simulink model "SecRwRtStLgrstUpwdDnwdCtrl"  (R2018b)
settings: Solver=FixedStepDiscrete  StartTime=0.0  StopTime=10.0  FixedStep=0.01  RelTol=1e-3
undefined symbols (not defined in the file or in its folder): KeSMSuMdMotFinshdTm_Val, KeSMSuMdRetryTm1_Val, KeSMSuModeReqDurgTm_Val, KeSMSwSecRwRtStLgrstUpwdDnwdEnTrigBitMask_Val
libraries: StCtrlLibBkRecln x1
settings Model: Creator=sn2xws  LastModifiedBy=sn55gm
settings Model: ModifiedHistory=|
  | 2024.10.14 V3.0.0 bitmask 更换变量接口
  | 25.7.7 V3.13.0 Md61 Md62新增Retry口
settings DataIOCC: SaveFormat=StructureWithTime
settings OptimizationCC: DefaultParameterBehavior=Inlined  EnhancedBackFolding=on  PassReuseOutputArgsAs=Individual arguments  ZeroExternalMemoryAtStartup=off  ZeroInternalMemoryAtStartup=off  OptimizeBlockOrder=speed  DifferentSizesBufferReuse=on  OptimizationCustomize=off
settings DebuggingCC: ParameterTunabilityLossMsg=error
settings ModelReferenceCC: ModelReferenceNumInstancesAllowed=Single
settings SFSimCC: MATLABDynamicMemAlloc=off
settings RTWCC: SystemTargetFile=autosar.tlc  GenCodeOnly=on  TemplateMakefile=ert_default_tmf  Description=AUTOSAR  GenerateReport=on  IncludeHyperlinkInReport=on  LaunchReport=on  GenerateTraceInfo=on  GenerateTraceReport=on  GenerateTraceReportSl=on  GenerateTraceReportSf=on  GenerateTraceReportEml=on
settings CodeAppCC: ForceParamTrailComments=on  IgnoreCustomStorageClasses=off  OperatorAnnotations=on  SimulinkDataObjDesc=on  SFDataObjDesc=on  InsertBlockDesc=on
settings STFCustomTargetCC: TargetLangStandard=C99 (ISO)  MultiwordLength=256  ParMdlRefBuildCompliant=on  CompOptLevelCompliant=on  IncludeMdlTerminateFcn=off  CombineOutputUpdateFcns=on  SuppressErrorStatus=on  ERTCustomFileBanners=on  SupportNonFinite=off  SupportComplex=off  SupportContinuousTime=off  SupportNonInlinedSFcns=off  RemoveResetFunc=on  MATLABClassNameForMDSCustomization=Simulink.SoftwareTarget.ERTCustomization  AutosarCompliant=on  UseToolchainInfoCompliant=on  LookupTableObjectStructAxisOrder=2,1,3,4,...  LUTObjectStructOrderEvenSpacing=Size,Table,Breakpoints  SystemTargetFile=autosar.tlc
settings ERTTargetCC: TargetLangStandard=C99 (ISO)  ConcurrentExecutionCompliant=off  IncludeMdlTerminateFcn=off  SuppressErrorStatus=on  SupportNonFinite=off  SupportComplex=off  ModelStepFunctionPrototypeControlCompliant=off  CPPClassGenCompliant=off  AutosarCompliant=on  LookupTableObjectStructAxisOrder=2,1,3,4,...  LUTObjectStructOrderEvenSpacing=Size,Table,Breakpoints  InlinedParameterPlacement=NonHierarchical  ERTCustomFileTemplate=example_file_process.tlc  ERTFilePackagingFormat=Compact

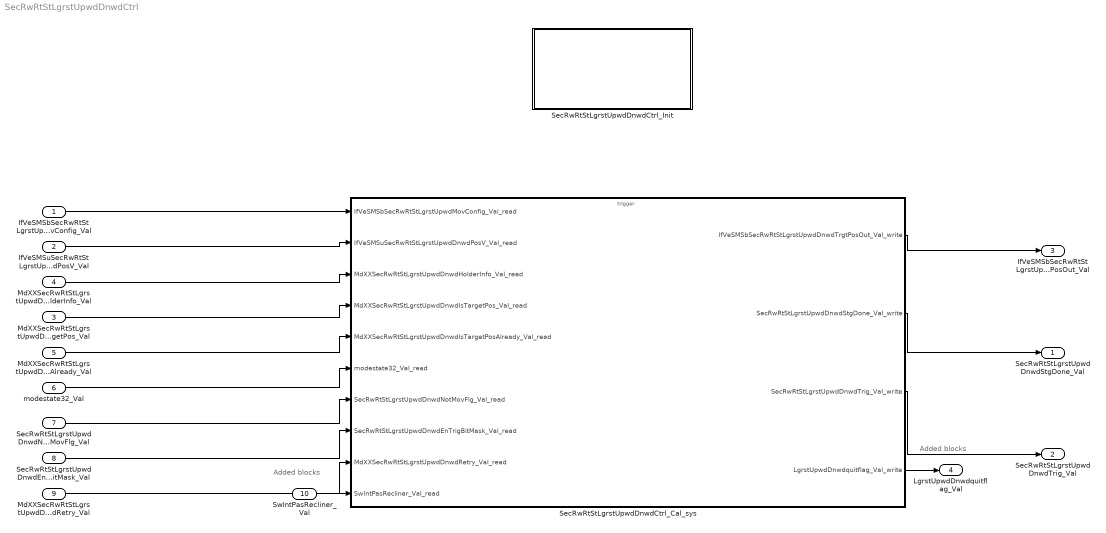
== system SecRwRtStLgrstUpwdDnwdCtrl ==
  note: Added blocks
  note: Added blocks
  IfVeSMSbSecRwRtStLgrstUpwdMovConfig_Val : Inport  OutDataTypeStr=boolean  PortDimensions=1
  IfVeSMSuSecRwRtStLgrstUpwdDnwdPosV_Val : Inport  Port=2  OutDataTypeStr=boolean  PortDimensions=1
  MdXXSecRwRtStLgrstUpwdDnwdIsTargetPos_Val : Inport  Port=3  OutDataTypeStr=uint32  PortDimensions=1
  MdXXSecRwRtStLgrstUpwdDnwdHolderInfo_Val : Inport  Port=4  OutDataTypeStr=uint32  PortDimensions=1
  MdXXSecRwRtStLgrstUpwdDnwdIsTargetPosAlready_Val : Inport  Port=5  OutDataTypeStr=uint32  PortDimensions=1
  modestate32_Val : Inport  Port=6  OutDataTypeStr=uint32  PortDimensions=1
  SecRwRtStLgrstUpwdDnwdNotMovFlg_Val : Inport  Port=7  OutDataTypeStr=boolean  PortDimensions=1
  SecRwRtStLgrstUpwdDnwdEnTrigBitMask_Val : Inport  Port=8  OutDataTypeStr=uint32  PortDimensions=1
  MdXXSecRwRtStLgrstUpwdDnwdRetry_Val : Inport  Port=9  OutDataTypeStr=uint32  PortDimensions=1
  SwIntPasRecliner_Val : Inport  Port=10  OutDataTypeStr=boolean  PortDimensions=1
  SecRwRtStLgrstUpwdDnwdCtrl_Cal_sys : Subsystem
  SecRwRtStLgrstUpwdDnwdCtrl_Init : Subsystem
  SecRwRtStLgrstUpwdDnwdStgDone_Val : Outport  OutDataTypeStr=boolean  PortDimensions=1
  SecRwRtStLgrstUpwdDnwdTrig_Val : Outport  Port=2  OutDataTypeStr=boolean  PortDimensions=1
  IfVeSMSbSecRwRtStLgrstUpwdDnwdTrgtPosOut_Val : Outport  Port=3  OutDataTypeStr=boolean  PortDimensions=1
  LgrstUpwdDnwdquitflag_Val : Outport  Port=4  OutDataTypeStr=boolean  PortDimensions=1
  wires:
  IfVeSMSbSecRwRtStLgrstUpwdMovConfig_Val/1 -> SecRwRtStLgrstUpwdDnwdCtrl_Cal_sys/1(IfVeSMSbSecRwRtStLgrstUpwdMovConfig_Val_read)
  IfVeSMSuSecRwRtStLgrstUpwdDnwdPosV_Val/1 -> SecRwRtStLgrstUpwdDnwdCtrl_Cal_sys/2(IfVeSMSuSecRwRtStLgrstUpwdDnwdPosV_Val_read)
  MdXXSecRwRtStLgrstUpwdDnwdIsTargetPos_Val/1 -> SecRwRtStLgrstUpwdDnwdCtrl_Cal_sys/4(MdXXSecRwRtStLgrstUpwdDnwdIsTargetPos_Val_read)
  MdXXSecRwRtStLgrstUpwdDnwdHolderInfo_Val/1 -> SecRwRtStLgrstUpwdDnwdCtrl_Cal_sys/3(MdXXSecRwRtStLgrstUpwdDnwdHolderInfo_Val_read)
  MdXXSecRwRtStLgrstUpwdDnwdIsTargetPosAlready_Val/1 -> SecRwRtStLgrstUpwdDnwdCtrl_Cal_sys/5(MdXXSecRwRtStLgrstUpwdDnwdIsTargetPosAlready_Val_read)
  modestate32_Val/1 -> SecRwRtStLgrstUpwdDnwdCtrl_Cal_sys/6(modestate32_Val_read)
  SecRwRtStLgrstUpwdDnwdNotMovFlg_Val/1 -> SecRwRtStLgrstUpwdDnwdCtrl_Cal_sys/7(SecRwRtStLgrstUpwdDnwdNotMovFlg_Val_read)
  SecRwRtStLgrstUpwdDnwdCtrl_Cal_sys/1(IfVeSMSbSecRwRtStLgrstUpwdDnwdTrgtPosOut_Val_write) -> IfVeSMSbSecRwRtStLgrstUpwdDnwdTrgtPosOut_Val/1
  SecRwRtStLgrstUpwdDnwdCtrl_Cal_sys/2(SecRwRtStLgrstUpwdDnwdStgDone_Val_write) -> SecRwRtStLgrstUpwdDnwdStgDone_Val/1
  SecRwRtStLgrstUpwdDnwdCtrl_Cal_sys/3(SecRwRtStLgrstUpwdDnwdTrig_Val_write) -> SecRwRtStLgrstUpwdDnwdTrig_Val/1
  SecRwRtStLgrstUpwdDnwdEnTrigBitMask_Val/1 -> SecRwRtStLgrstUpwdDnwdCtrl_Cal_sys/8(SecRwRtStLgrstUpwdDnwdEnTrigBitMask_Val_read)
  MdXXSecRwRtStLgrstUpwdDnwdRetry_Val/1 -> SecRwRtStLgrstUpwdDnwdCtrl_Cal_sys/9(MdXXSecRwRtStLgrstUpwdDnwdRetry_Val_read)
  SecRwRtStLgrstUpwdDnwdCtrl_Cal_sys/4(LgrstUpwdDnwdquitflag_Val_write) -> LgrstUpwdDnwdquitflag_Val/1
  SwIntPasRecliner_Val/1 -> SecRwRtStLgrstUpwdDnwdCtrl_Cal_sys/10(SwIntPasRecliner_Val_read)

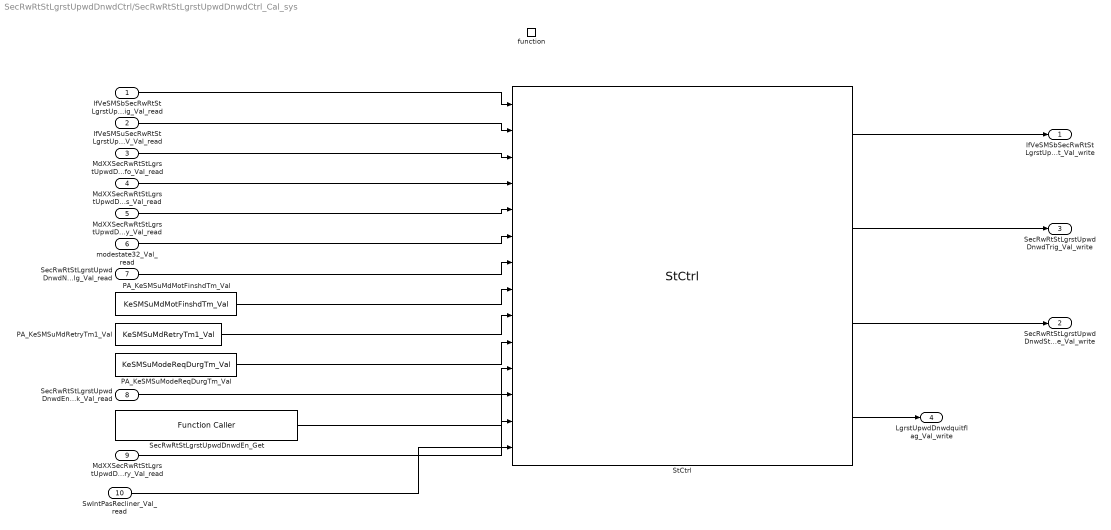
== system SecRwRtStLgrstUpwdDnwdCtrl/SecRwRtStLgrstUpwdDnwdCtrl_Cal_sys ==
  IfVeSMSbSecRwRtStLgrstUpwdMovConfig_Val_read : Inport
  IfVeSMSuSecRwRtStLgrstUpwdDnwdPosV_Val_read : Inport  Port=2
  MdXXSecRwRtStLgrstUpwdDnwdHolderInfo_Val_read : Inport  Port=3
  MdXXSecRwRtStLgrstUpwdDnwdIsTargetPos_Val_read : Inport  Port=4
  MdXXSecRwRtStLgrstUpwdDnwdIsTargetPosAlready_Val_read : Inport  Port=5
  modestate32_Val_read : Inport  Port=6
  SecRwRtStLgrstUpwdDnwdNotMovFlg_Val_read : Inport  Port=7
  SecRwRtStLgrstUpwdDnwdEnTrigBitMask_Val_read : Inport  Port=8
  MdXXSecRwRtStLgrstUpwdDnwdRetry_Val_read : Inport  Port=9
  SwIntPasRecliner_Val_read : Inport  Port=10
  function : TriggerPort  TriggerType=function-call  IsSimulinkFunction=on  FunctionName=SecRwRtStLgrstUpwdDnwdCtrl_Cal  VariantControl=(inherit)
  PA_KeSMSuMdMotFinshdTm_Val : Constant  Value=KeSMSuMdMotFinshdTm_Val
  PA_KeSMSuMdRetryTm1_Val : Constant  Value=KeSMSuMdRetryTm1_Val
  PA_KeSMSuModeReqDurgTm_Val : Constant  Value=KeSMSuModeReqDurgTm_Val
  SecRwRtStLgrstUpwdDnwdEn_Get : FunctionCaller  FunctionPrototype=data = SecRwRtStLgrstUpwdDnwdEn_Get()  OutputArgumentSpecifications=uint32(1)
  StCtrl : StCtrlLibBkRecln/StCtrl  SystemSampleTime=-1
  IfVeSMSbSecRwRtStLgrstUpwdDnwdTrgtPosOut_Val_write : Outport
      settings: EnsureOutportIsVirtual=on
  SecRwRtStLgrstUpwdDnwdStgDone_Val_write : Outport  Port=2
      settings: EnsureOutportIsVirtual=on
  SecRwRtStLgrstUpwdDnwdTrig_Val_write : Outport  Port=3
      settings: EnsureOutportIsVirtual=on
  LgrstUpwdDnwdquitflag_Val_write : Outport  Port=4
      settings: EnsureOutportIsVirtual=on
  wires:
  StCtrl/3 -> SecRwRtStLgrstUpwdDnwdStgDone_Val_write/1
  StCtrl/2 -> SecRwRtStLgrstUpwdDnwdTrig_Val_write/1
  StCtrl/1 -> IfVeSMSbSecRwRtStLgrstUpwdDnwdTrgtPosOut_Val_write/1
  SecRwRtStLgrstUpwdDnwdEnTrigBitMask_Val_read/1 -> StCtrl/11
  SecRwRtStLgrstUpwdDnwdEn_Get/1 -> StCtrl/12
  PA_KeSMSuMdMotFinshdTm_Val/1 -> StCtrl/8
  PA_KeSMSuModeReqDurgTm_Val/1 -> StCtrl/10
  PA_KeSMSuMdRetryTm1_Val/1 -> StCtrl/9
  modestate32_Val_read/1 -> StCtrl/6
  SecRwRtStLgrstUpwdDnwdNotMovFlg_Val_read/1 -> StCtrl/7
  MdXXSecRwRtStLgrstUpwdDnwdIsTargetPosAlready_Val_read/1 -> StCtrl/5
  MdXXSecRwRtStLgrstUpwdDnwdIsTargetPos_Val_read/1 -> StCtrl/4
  MdXXSecRwRtStLgrstUpwdDnwdHolderInfo_Val_read/1 -> StCtrl/3
  IfVeSMSuSecRwRtStLgrstUpwdDnwdPosV_Val_read/1 -> StCtrl/2
  IfVeSMSbSecRwRtStLgrstUpwdMovConfig_Val_read/1 -> StCtrl/1
  MdXXSecRwRtStLgrstUpwdDnwdRetry_Val_read/1 -> StCtrl/13
  StCtrl/4 -> LgrstUpwdDnwdquitflag_Val_write/1
  SwIntPasRecliner_Val_read/1 -> StCtrl/14

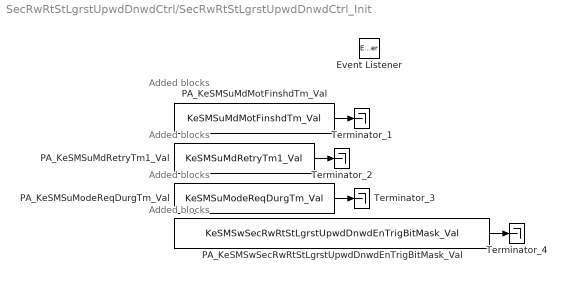
== system SecRwRtStLgrstUpwdDnwdCtrl/SecRwRtStLgrstUpwdDnwdCtrl_Init ==
  note: Added blocks
  note: Added blocks
  note: Added blocks
  note: Added blocks
  Event Listener : EventListener  EventName=reset
  PA_KeSMSuMdMotFinshdTm_Val : Constant  Value=KeSMSuMdMotFinshdTm_Val
  PA_KeSMSuMdRetryTm1_Val : Constant  Value=KeSMSuMdRetryTm1_Val
  PA_KeSMSuModeReqDurgTm_Val : Constant  Value=KeSMSuModeReqDurgTm_Val
  PA_KeSMSwSecRwRtStLgrstUpwdDnwdEnTrigBitMask_Val : Constant  Value=KeSMSwSecRwRtStLgrstUpwdDnwdEnTrigBitMask_Val
  Terminator_{1..4} (4 alike) : Terminator
  wires:
  PA_KeSMSuMdMotFinshdTm_Val/1 -> Terminator_1/1
  PA_KeSMSuMdRetryTm1_Val/1 -> Terminator_2/1
  PA_KeSMSuModeReqDurgTm_Val/1 -> Terminator_3/1
  PA_KeSMSwSecRwRtStLgrstUpwdDnwdEnTrigBitMask_Val/1 -> Terminator_4/1
